simulink model "singleareamultiitae"  (R2014a)
settings: Solver=ode45  StartTime=0.0  StopTime=60  RelTol=1e-3
libraries: simulink x1
settings Model: Creator=Admin1  LastModifiedBy=Admin

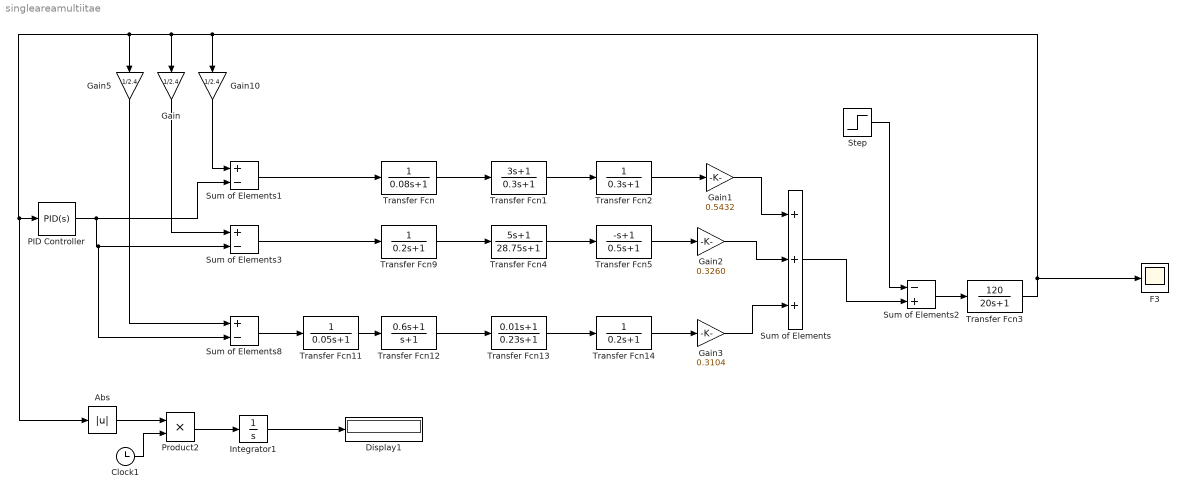
== system singleareamultiitae ==
  Abs : Abs
  Clock1 : Clock
  Display1 : Display
  F3 : Scope
  Gain : Gain  Gain=1/2.4
  Gain1 : Gain  Gain=0.5432
  Gain10 : Gain  Gain=1/2.4
  Gain2 : Gain  Gain=0.3260
  Gain3 : Gain  Gain=0.3104
  Gain5 : Gain  Gain=1/2.4
  Integrator1 : Integrator
  PID Controller : simulink/Continuous/PID Controller  Controller=PID  TimeDomain=Continuous-time  SampleTime=1  IntegratorMethod=Forward Euler  FilterMethod=Forward Euler  Form=Parallel  P=0.6  I=0.364  D=0.1  N=100  InitialConditionSource=internal  InitialConditionForIntegrator=0  InitialConditionForFilter=0  ExternalReset=none  LimitOutput=off  UpperSaturationLimit=inf  LowerSaturationLimit=-inf  LinearizeAsGain=on  AntiWindupMode=none  Kb=1  TrackingMode=off  Kt=1  PParamMin=[]  PParamMax=[]  IParamMin=[]  IParamMax=[]  DParamMin=[]  DParamMax=[]  NParamMin=[]  NParamMax=[]  KbParamMin=[]  KbParamMax=[]  KtParamMin=[]  KtParamMax=[]  POutMin=[]  POutMax=[]  IOutMin=[]  IOutMax=[]  DOutMin=[]  DOutMax=[]  NOutMin=[]  NOutMax=[]  KbOutMin=[]  KbOutMax=[]  KtOutMin=[]  KtOutMax=[]  IntegratorOutMin=[]  IntegratorOutMax=[]  FilterOutMin=[]  FilterOutMax=[]  SumOutMin=[]  SumOutMax=[]  SumI1OutMin=[]  SumI1OutMax=[]  SumI2OutMin=[]  SumI2OutMax=[]  SumI3OutMin=[]  SumI3OutMax=[]  SumDOutMin=[]  SumDOutMax=[]  SaturationOutMin=[]  SaturationOutMax=[]  IntegratorContinuousStateAttributes=''  IntegratorStateMustResolveToSignalObject=off  IntegratorRTWStateStorageClass=Auto  FilterContinuousStateAttributes=''  FilterStateMustResolveToSignalObject=off  FilterRTWStateStorageClass=Auto
  Product2 : Product  RndMeth=Zero
  Step : Step  After=0.01  SampleTime=0
  Sum of Elements : Sum  Inputs=+++
  Sum of Elements1 : Sum  Inputs=+-
  Sum of Elements2 : Sum  Inputs=-+
  Sum of Elements3 : Sum  Inputs=+-
  Sum of Elements8 : Sum  Inputs=+-
  Transfer Fcn : TransferFcn  Denominator=[0.08 1]
  Transfer Fcn1 : TransferFcn  Numerator=[3 1]  Denominator=[0.3 1]
  Transfer Fcn11 : TransferFcn  Denominator=[0.05 1]
  Transfer Fcn12 : TransferFcn  Numerator=[0.6 1]  Denominator=[1 1]
  Transfer Fcn13 : TransferFcn  Numerator=[0.01 1]  Denominator=[0.23 1]
  Transfer Fcn14 : TransferFcn  Denominator=[0.2 1]
  Transfer Fcn2 : TransferFcn  Numerator=[ 1]  Denominator=[0.3 1]
  Transfer Fcn3 : TransferFcn  Numerator=[120]  Denominator=[20 1]
  Transfer Fcn4 : TransferFcn  Numerator=[5 1]  Denominator=[28.75 1]
  Transfer Fcn5 : TransferFcn  Numerator=[-1 1]  Denominator=[0.5 1]
  Transfer Fcn9 : TransferFcn  Denominator=[0.2 1]
  wires:
  Sum of Elements8/1 -> Transfer Fcn11/1
  Transfer Fcn11/1 -> Transfer Fcn12/1
  Transfer Fcn12/1 -> Transfer Fcn13/1
  Transfer Fcn13/1 -> Transfer Fcn14/1
  Transfer Fcn/1 -> Transfer Fcn1/1
  Transfer Fcn1/1 -> Transfer Fcn2/1
  Sum of Elements1/1 -> Transfer Fcn/1
  Transfer Fcn2/1 -> Gain1/1
  Gain1/1 -> Sum of Elements/1
  Sum of Elements3/1 -> Transfer Fcn9/1
  Transfer Fcn9/1 -> Transfer Fcn4/1
  Transfer Fcn4/1 -> Transfer Fcn5/1
  Transfer Fcn5/1 -> Gain2/1
  Gain2/1 -> Sum of Elements/2
  Gain3/1 -> Sum of Elements/3
  Transfer Fcn14/1 -> Gain3/1
  Step/1 -> Sum of Elements2/1
  Sum of Elements/1 -> Sum of Elements2/2
  Sum of Elements2/1 -> Transfer Fcn3/1
  Gain10/1 -> Sum of Elements1/1
  Gain/1 -> Sum of Elements3/1
  Gain5/1 -> Sum of Elements8/1
  Transfer Fcn3/1 -> F3/1, Gain10/1, Gain/1, Gain5/1, Abs/1, PID Controller/1
  PID Controller/1 -> Sum of Elements8/2, Sum of Elements3/2, Sum of Elements1/2
  Abs/1 -> Product2/1
  Clock1/1 -> Product2/2
  Product2/1 -> Integrator1/1
  Integrator1/1 -> Display1/1
